simulink model "MSupGesamt"  (R2018b)
settings: Solver=FixedStepDiscrete  StartTime=0.0  StopTime=10.0  RelTol=1e-3  EnableMultiTasking=on
libraries: commutil2 x12, c280xlib x10, c2833xlib x9, c2000lib x1
(part 1 of 2)
settings Model: ExtModeTrigDuration=8  Creator=User  LastModifiedBy=ulvqy
settings SolverCC: AutoInsertRateTranBlk=on
settings DataIOCC: LimitDataPoints=on  SaveFormat=Array  SaveOutput=off  SaveTime=off
settings OptimizationCC: DefaultUnderspecifiedDataType=single  ExpressionDepthLimit=2147483647  LifeSpan=1  MaxStackSize=512
settings DebuggingCC: UnderspecifiedInitializationDetection=Classic  MergeDetectMultiDrivingBlocksExec=none  SolverPrmCheckMsg=warning  StateNameClashWarn=warning  SFUnexpectedBacktrackingDiag=warning  SFNoUnconditionalDefaultTransitionDiag=warning  SFExecutionAtInitializationDiag=none
settings HardwareCC: ProdBitPerChar=16  ProdBitPerInt=16  ProdBitPerPointer=32  ProdBitPerSizeT=32  ProdBitPerPtrDiffT=32  ProdLargestAtomicInteger=Integer  ProdLargestAtomicFloat=None  ProdWordSize=16  ProdLongLongMode=on  ProdHWDeviceType=Texas Instruments->C2000  TargetBitPerChar=16  TargetBitPerInt=16  TargetLargestAtomicInteger=Integer  TargetIntDivRoundTo=Zero  TargetEndianess=LittleEndian  TargetWordSize=16  TargetHWDeviceType=Texas Instruments->C2000  ProdEqTarget=off
settings ModelReferenceCC: PropagateSignalLabelsOutOfModel=off
settings SFSimCC: SimCustomSourceCode="#include \"i2c_reset.c\""  SimCustomHeaderCode="#include \"i2c_reset.h\""  SimUseLocalCustomCode=off  MATLABDynamicMemAlloc=off
settings RTWCC: SystemTargetFile=ert.tlc  HardwareBoard=TI Delfino F2833x  TemplateMakefile=ert_default_tmf  RTWUseLocalCustomCode=off  RTWUseSimCustomCode=on  CustomSourceCode="#include \"i2c_reset.c\""  CustomHeaderCode="#include \"i2c_reset.h\""  Toolchain=Texas Instruments Code Composer Studio (C2000)
settings CodeAppCC: IgnoreCustomStorageClasses=off  CustomSymbolStrType=$N$R$M  StateflowObjectComments=on  InternalIdentifier=Classic
settings ERTTargetCC: CodeReplacementLibrary=TI C28x  MultiwordLength=2048  ParMdlRefBuildCompliant=off  CPPClassGenCompliant=off  ConvertIfToSwitch=off  SuppressUnreachableDefaultCases=off
settings ConfigComp: CovMetricSettings=dw  CovHtmlReporting=on  CovSaveCumulativeToWorkspaceVar=on  CovSaveSingleToWorkspaceVar=on  CovExternalEMLEnable=off

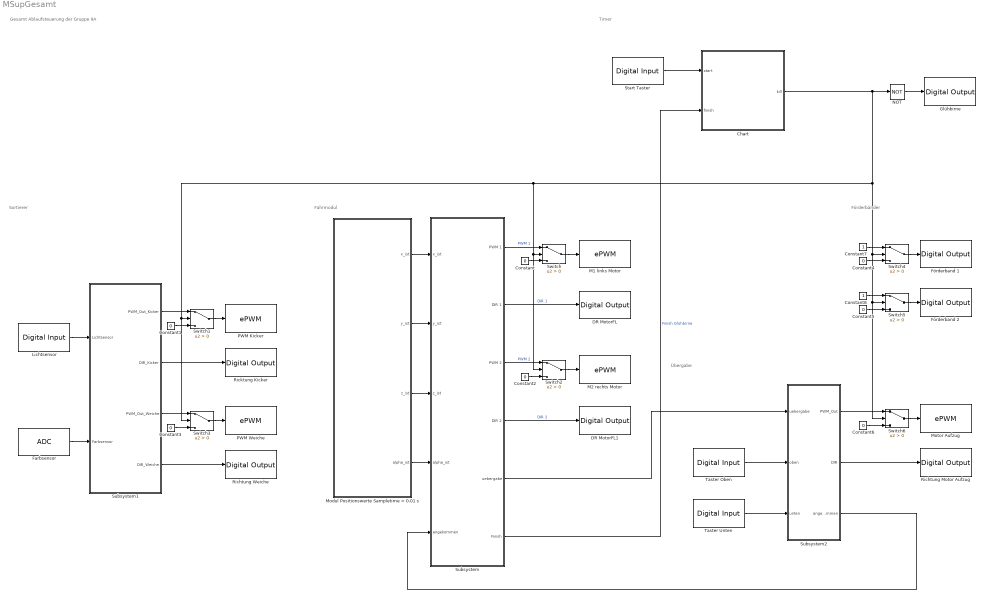
== system MSupGesamt ==
  note: Gesamt Ablaufsteuerung der Gruppe 9A
  note: Übergabe
  note: Timer
  note: Förderbänder
  note: Fahrmodul
  note: Sortierer
  Chart : Stateflow chart  TreatAsAtomicUnit=on
  Constant{,1..6} (7 alike) : Constant  Value=0
  Constant7 : Constant
  Constant8 : Constant
  DR MotorFL : c2833xlib/Digital Output  GPIO_Number=GPIO16~GPIO23  GPIO_Bit0=off  GPIO_BIT0_Toggle=off  GPIO_Bit1=off  GPIO_BIT1_Toggle=off  GPIO_Bit2=off  GPIO_BIT2_Toggle=off  GPIO_Bit3=off  GPIO_BIT3_Toggle=off  GPIO_Bit4=off  GPIO_BIT4_Toggle=off  GPIO_Bit5=on  GPIO_BIT5_Toggle=off  GPIO_Bit6=off  GPIO_BIT6_Toggle=off  GPIO_Bit7=off  GPIO_BIT7_Toggle=off
      settings: SourceProductName=Embedded Coder Support Package for Texas Instruments C2000 Processors  SourceProductBaseCode=TIC2000
  DR MotorFL1 : c2833xlib/Digital Output  GPIO_Number=GPIO16~GPIO23  GPIO_Bit0=off  GPIO_BIT0_Toggle=off  GPIO_Bit1=off  GPIO_BIT1_Toggle=off  GPIO_Bit2=off  GPIO_BIT2_Toggle=off  GPIO_Bit3=off  GPIO_BIT3_Toggle=off  GPIO_Bit4=on  GPIO_BIT4_Toggle=off  GPIO_Bit5=off  GPIO_BIT5_Toggle=off  GPIO_Bit6=off  GPIO_BIT6_Toggle=off  GPIO_Bit7=off  GPIO_BIT7_Toggle=off
      settings: SourceProductName=Embedded Coder Support Package for Texas Instruments C2000 Processors  SourceProductBaseCode=TIC2000
  Farbsensor : c280xlib/ADC  useModule=A  useMode=Sequential  sourceSOC=Software  sourceSOC1=Software  sourceSOC2=ePWMxB  xint2_ADCSOC=31  Ts=0.00002  dType=double  postInterrupt=off  numConversionsSingle=1  numConversionsDouble=1  conv0=ADCINA0  conv1=ADCINA1  conv2=ADCINA2  conv3=ADCINA3  conv4=ADCINA4  conv5=ADCINA5  conv6=ADCINA6  conv7=ADCINA7  conv8=ADCINB0  conv9=ADCINB1  conv10=ADCINB2  conv11=ADCINB3  conv12=ADCINB4  conv13=ADCINB5  conv14=ADCINB6  conv15=ADCINB7  convAB0=ADCINA0 and ADCINB0  convAB1=ADCINA1 and ADCINB1  convAB2=ADCINA2 and ADCINB2  convAB3=ADCINA3 and ADCINB3  convAB4=ADCINA4 and ADCINB4  convAB5=ADCINA5 and ADCINB5  convAB6=ADCINA6 and ADCINB6  convAB7=ADCINA7 and ADCINB7  convA0=ADCINA2  convA1=ADCINA1  convA2=ADCINA2  convA3=ADCINA3  convA4=ADCINA5  convA5=ADCINA5  convA6=ADCINA6  convA7=ADCINA7  convB0=ADCINB0  convB1=ADCINB1  convB2=ADCINB2  convB3=ADCINB3  convB4=ADCINB4  convB5=ADCINB5  convB6=ADCINB6  convB7=ADCINB7  c28xmultiPort=off  endma=off  chdma=1
      settings: SourceProductName=Embedded Coder Support Package for Texas Instruments C2000 Processors  SourceProductBaseCode=TIC2000
  Förderband 1 : c2833xlib/Digital Output  GPIO_Number=GPIO56~GPIO63  GPIO_Bit0=off  GPIO_BIT0_Toggle=off  GPIO_Bit1=off  GPIO_BIT1_Toggle=off  GPIO_Bit2=on  GPIO_BIT2_Toggle=off  GPIO_Bit3=off  GPIO_BIT3_Toggle=off  GPIO_Bit4=off  GPIO_BIT4_Toggle=off  GPIO_Bit5=off  GPIO_BIT5_Toggle=off  GPIO_Bit6=off  GPIO_BIT6_Toggle=off  GPIO_Bit7=off  GPIO_BIT7_Toggle=off
      settings: SourceProductName=Embedded Coder Support Package for Texas Instruments C2000 Processors  SourceProductBaseCode=TIC2000
  Förderband 2 : c2833xlib/Digital Output  GPIO_Number=GPIO56~GPIO63  GPIO_Bit0=off  GPIO_BIT0_Toggle=off  GPIO_Bit1=off  GPIO_BIT1_Toggle=off  GPIO_Bit2=off  GPIO_BIT2_Toggle=off  GPIO_Bit3=off  GPIO_BIT3_Toggle=off  GPIO_Bit4=off  GPIO_BIT4_Toggle=off  GPIO_Bit5=on  GPIO_BIT5_Toggle=off  GPIO_Bit6=off  GPIO_BIT6_Toggle=off  GPIO_Bit7=off  GPIO_BIT7_Toggle=off
      settings: SourceProductName=Embedded Coder Support Package for Texas Instruments C2000 Processors  SourceProductBaseCode=TIC2000
  Glühbirne : c2833xlib/Digital Output  GPIO_Number=GPIO56~GPIO63  GPIO_Bit0=off  GPIO_BIT0_Toggle=off  GPIO_Bit1=off  GPIO_BIT1_Toggle=off  GPIO_Bit2=off  GPIO_BIT2_Toggle=off  GPIO_Bit3=off  GPIO_BIT3_Toggle=off  GPIO_Bit4=on  GPIO_BIT4_Toggle=off  GPIO_Bit5=off  GPIO_BIT5_Toggle=off  GPIO_Bit6=off  GPIO_BIT6_Toggle=off  GPIO_Bit7=off  GPIO_BIT7_Toggle=off
      settings: SourceProductName=Embedded Coder Support Package for Texas Instruments C2000 Processors  SourceProductBaseCode=TIC2000
  Lichtsensor : c280xlib/Digital Input  GPIO_Number=GPIO24~GPIO31  GPIO_Bit0=off  GPIO_Bit1=on  GPIO_Bit2=off  GPIO_Bit3=off  GPIO_Bit4=off  GPIO_Bit5=off  GPIO_Bit6=off  GPIO_Bit7=off  sampleTime=0.1  dataType=auto  GPIO_Bit0_Qualification=Sync to SYSCLKOUT  GPIO_Bit1_Qualification=Sync to SYSCLKOUT  GPIO_Bit2_Qualification=Sync to SYSCLKOUT  GPIO_Bit3_Qualification=Sync to SYSCLKOUT  GPIO_Bit4_Qualification=Sync to SYSCLKOUT  GPIO_Bit5_Qualification=Sync to SYSCLKOUT  GPIO_Bit6_Qualification=Sync to SYSCLKOUT  GPIO_Bit7_Qualification=Sync to SYSCLKOUT  Qualification_Period=-1
      settings: SourceProductName=Embedded Coder Support Package for Texas Instruments C2000 Processors  SourceProductBaseCode=TIC2000
  M1 links Motor : c280xlib/ePWM  checkMode=off  useModule=ePWM2  periodUnits=Clock cycles  timerSource=Specify via dialog  timerPeriod_clk=64000  timerPeriod_sec=0.0001  tbshadow=Counter equals to zero  countingMode=Up  phaseActiveEnable=Disable  phaseDirection=Count down after sync  phaseActive=0  synchronizationEnable=off  synchronizationOption=Disable  clockPrescale=1  HSclockPrescale=1  ePWMxAStatus=on  CMPAUnits=Clock cycles  CMPASource=Specify via dialog  CMPAValue_per=50  CMPAValue_clk=32000  enCMPAshadow=Counter equals to zero  ePWMxAactionLogic1=Set  ePWMxAactionLogic2=Clear  ePWMxAactionLogic3=Clear  ePWMxAactionLogic4=Set  ePWMxAactionLogic5=Do nothing  ePWMxAactionLogic6=Do nothing  ePWMxALoadMode=Load on counter equals to zero (CTR=Zero)  ePWMxACSFenable=off  ePWMxACSFvalue=Forcing disable  ePWMxASFreload=Zero  enHRPWM=off  HRPWM_LoadMode=Counter equals to zero (CTR=ZERO)  HRPWM_CTLMode=Phase control mode  HRPWM_EDGMode=Both edge  enSFO=on  ePWMxBStatus=on  CMPBUnits=Percentages  CMPBSource=Input port  CMPBValue_per=0  CMPBValue_clk=32000  enCMPBshadow=Counter equals to zero  ePWMxBactionLogic1=Do nothing  ePWMxBactionLogic2=Set  ePWMxBactionLogic3=Do nothing  ePWMxBactionLogic4=Do nothing  ePWMxBactionLogic5=Clear  ePWMxBactionLogic6=Do nothing  ePWMxBLoadMode=Load on counter equals to zero (CTR=Zero)  ePWMxBCSFenable=off  ePWMxBCSFvalue=Forcing disable  ePWMxBSFreload=Zero  enableDBePWMxA=off  enableDBePWMxB=off  DBpolarity=Active high (AH)  DBedgeDelay=Positive  DBSource_ePWMxA=ePWMxA  DBSource_ePWMxB=ePWMxA  DBperiodSource=Specify via dialog  REDperiod=0  FEDperiod=0  adcstartModuleA=off  adcrequestEventA=First event  adcstartEventA=Counter equals to zero (CTR=Zero)  adcstartModuleB=off  adcrequestEventB=First event  adcstartEventB=Counter equals to zero (CTR=Zero)  intEn=off  intPrd=First event  intSel=Counter equals to zero (CTR=Zero)  chopperEnable=off  chopperFrequency=1  chopperFirstwidth=1  chopperDuty=12.5%  tripZonesource=Specify via dialog  tzselOSHT1=off  tzselOSHT2=off  tzselOSHT3=off  tzselOSHT4=off  tzselOSHT5=off  tzselOSHT6=off  tzselCBC1=off  tzselCBC2=off  tzselCBC3=off  tzselCBC4=off  tzselCBC5=off  tzselCBC6=off  enTzOstIntr=off  enTzCbcIntr=off  ePWMxAforced=No action  ePWMxBforced=No action  timerPeriod=-1  ePWMxAValue=0  ePWMxBValue=0  tripZoneoption=One-shot trip (OSHT)
      settings: SourceProductName=Embedded Coder Support Package for Texas Instruments C2000 Processors  SourceProductBaseCode=TIC2000
  M2 rechts Motor : c280xlib/ePWM  checkMode=off  useModule=ePWM1  periodUnits=Clock cycles  timerSource=Specify via dialog  timerPeriod_clk=64000  timerPeriod_sec=0.0001  tbshadow=Counter equals to zero  countingMode=Up  phaseActiveEnable=Disable  phaseDirection=Count down after sync  phaseActive=0  synchronizationEnable=off  synchronizationOption=Disable  clockPrescale=1  HSclockPrescale=1  ePWMxAStatus=on  CMPAUnits=Clock cycles  CMPASource=Specify via dialog  CMPAValue_per=50  CMPAValue_clk=32000  enCMPAshadow=Counter equals to zero  ePWMxAactionLogic1=Set  ePWMxAactionLogic2=Clear  ePWMxAactionLogic3=Clear  ePWMxAactionLogic4=Set  ePWMxAactionLogic5=Do nothing  ePWMxAactionLogic6=Do nothing  ePWMxALoadMode=Load on counter equals to zero (CTR=Zero)  ePWMxACSFenable=off  ePWMxACSFvalue=Forcing disable  ePWMxASFreload=Zero  enHRPWM=off  HRPWM_LoadMode=Counter equals to zero (CTR=ZERO)  HRPWM_CTLMode=Phase control mode  HRPWM_EDGMode=Both edge  enSFO=on  ePWMxBStatus=on  CMPBUnits=Percentages  CMPBSource=Input port  CMPBValue_per=0  CMPBValue_clk=32000  enCMPBshadow=Counter equals to zero  ePWMxBactionLogic1=Do nothing  ePWMxBactionLogic2=Set  ePWMxBactionLogic3=Do nothing  ePWMxBactionLogic4=Do nothing  ePWMxBactionLogic5=Clear  ePWMxBactionLogic6=Do nothing  ePWMxBLoadMode=Load on counter equals to zero (CTR=Zero)  ePWMxBCSFenable=off  ePWMxBCSFvalue=Forcing disable  ePWMxBSFreload=Zero  enableDBePWMxA=off  enableDBePWMxB=off  DBpolarity=Active high (AH)  DBedgeDelay=Positive  DBSource_ePWMxA=ePWMxA  DBSource_ePWMxB=ePWMxA  DBperiodSource=Specify via dialog  REDperiod=0  FEDperiod=0  adcstartModuleA=off  adcrequestEventA=First event  adcstartEventA=Counter equals to zero (CTR=Zero)  adcstartModuleB=off  adcrequestEventB=First event  adcstartEventB=Counter equals to zero (CTR=Zero)  intEn=off  intPrd=First event  intSel=Counter equals to zero (CTR=Zero)  chopperEnable=off  chopperFrequency=1  chopperFirstwidth=1  chopperDuty=12.5%  tripZonesource=Specify via dialog  tzselOSHT1=off  tzselOSHT2=off  tzselOSHT3=off  tzselOSHT4=off  tzselOSHT5=off  tzselOSHT6=off  tzselCBC1=off  tzselCBC2=off  tzselCBC3=off  tzselCBC4=off  tzselCBC5=off  tzselCBC6=off  enTzOstIntr=off  enTzCbcIntr=off  ePWMxAforced=No action  ePWMxBforced=No action  timerPeriod=-1  ePWMxAValue=0  ePWMxBValue=0  tripZoneoption=One-shot trip (OSHT)
      settings: SourceProductName=Embedded Coder Support Package for Texas Instruments C2000 Processors  SourceProductBaseCode=TIC2000
  Modul Positionswerte Sampletime = 0.01 s : Subsystem
  Motor Aufzug : c280xlib/ePWM  checkMode=off  useModule=ePWM3  periodUnits=Clock cycles  timerSource=Specify via dialog  timerPeriod_clk=64000  timerPeriod_sec=0.0001  tbshadow=Counter equals to zero  countingMode=Up  phaseActiveEnable=Disable  phaseDirection=Count down after sync  phaseActive=0  synchronizationEnable=off  synchronizationOption=Disable  clockPrescale=1  HSclockPrescale=1  ePWMxAStatus=on  CMPAUnits=Clock cycles  CMPASource=Specify via dialog  CMPAValue_per=50  CMPAValue_clk=32000  enCMPAshadow=Counter equals to zero  ePWMxAactionLogic1=Set  ePWMxAactionLogic2=Clear  ePWMxAactionLogic3=Clear  ePWMxAactionLogic4=Set  ePWMxAactionLogic5=Do nothing  ePWMxAactionLogic6=Do nothing  ePWMxALoadMode=Load on counter equals to zero (CTR=Zero)  ePWMxACSFenable=off  ePWMxACSFvalue=Forcing disable  ePWMxASFreload=Zero  enHRPWM=off  HRPWM_LoadMode=Counter equals to zero (CTR=ZERO)  HRPWM_CTLMode=Phase control mode  HRPWM_EDGMode=Both edge  enSFO=on  ePWMxBStatus=on  CMPBUnits=Percentages  CMPBSource=Input port  CMPBValue_per=0  CMPBValue_clk=32000  enCMPBshadow=Counter equals to zero  ePWMxBactionLogic1=Do nothing  ePWMxBactionLogic2=Set  ePWMxBactionLogic3=Do nothing  ePWMxBactionLogic4=Do nothing  ePWMxBactionLogic5=Clear  ePWMxBactionLogic6=Do nothing  ePWMxBLoadMode=Load on counter equals to zero (CTR=Zero)  ePWMxBCSFenable=off  ePWMxBCSFvalue=Forcing disable  ePWMxBSFreload=Zero  enableDBePWMxA=off  enableDBePWMxB=off  DBpolarity=Active high (AH)  DBedgeDelay=Positive  DBSource_ePWMxA=ePWMxA  DBSource_ePWMxB=ePWMxA  DBperiodSource=Specify via dialog  REDperiod=0  FEDperiod=0  adcstartModuleA=off  adcrequestEventA=First event  adcstartEventA=Counter equals to zero (CTR=Zero)  adcstartModuleB=off  adcrequestEventB=First event  adcstartEventB=Counter equals to zero (CTR=Zero)  intEn=off  intPrd=First event  intSel=Counter equals to zero (CTR=Zero)  chopperEnable=off  chopperFrequency=1  chopperFirstwidth=1  chopperDuty=12.5%  tripZonesource=Specify via dialog  tzselOSHT1=off  tzselOSHT2=off  tzselOSHT3=off  tzselOSHT4=off  tzselOSHT5=off  tzselOSHT6=off  tzselCBC1=off  tzselCBC2=off  tzselCBC3=off  tzselCBC4=off  tzselCBC5=off  tzselCBC6=off  enTzOstIntr=off  enTzCbcIntr=off  ePWMxAforced=No action  ePWMxBforced=No action  timerPeriod=-1  ePWMxAValue=0  ePWMxBValue=0  tripZoneoption=One-shot trip (OSHT)
      settings: SourceProductName=Embedded Coder Support Package for Texas Instruments C2000 Processors  SourceProductBaseCode=TIC2000
  NOT : Logic  Operator=NOT  IconShape=distinctive  AllPortsSameDT=off  OutDataTypeStr=boolean
  PWM Kicker : c280xlib/ePWM  checkMode=off  useModule=ePWM5  periodUnits=Clock cycles  timerSource=Specify via dialog  timerPeriod_clk=64000  timerPeriod_sec=0.0001  tbshadow=Counter equals to zero  countingMode=Up  phaseActiveEnable=Disable  phaseDirection=Count down after sync  phaseActive=0  synchronizationEnable=off  synchronizationOption=Disable  clockPrescale=1  HSclockPrescale=1  ePWMxAStatus=off  CMPAUnits=Clock cycles  CMPASource=Specify via dialog  CMPAValue_per=50  CMPAValue_clk=32000  enCMPAshadow=Counter equals to zero  ePWMxAactionLogic1=Do nothing  ePWMxAactionLogic2=Clear  ePWMxAactionLogic3=Set  ePWMxAactionLogic4=Do nothing  ePWMxAactionLogic5=Do nothing  ePWMxAactionLogic6=Do nothing  ePWMxALoadMode=Load on counter equals to zero (CTR=Zero)  ePWMxACSFenable=off  ePWMxACSFvalue=Forcing disable  ePWMxASFreload=Zero  enHRPWM=off  HRPWM_LoadMode=Counter equals to zero (CTR=ZERO)  HRPWM_CTLMode=Phase control mode  HRPWM_EDGMode=Both edge  enSFO=on  ePWMxBStatus=on  CMPBUnits=Percentages  CMPBSource=Input port  CMPBValue_per=0  CMPBValue_clk=32000  enCMPBshadow=Counter equals to zero  ePWMxBactionLogic1=Do nothing  ePWMxBactionLogic2=Set  ePWMxBactionLogic3=Do nothing  ePWMxBactionLogic4=Do nothing  ePWMxBactionLogic5=Clear  ePWMxBactionLogic6=Do nothing  ePWMxBLoadMode=Load on counter equals to zero (CTR=Zero)  ePWMxBCSFenable=off  ePWMxBCSFvalue=Forcing disable  ePWMxBSFreload=Zero  enableDBePWMxA=off  enableDBePWMxB=off  DBpolarity=Active high (AH)  DBedgeDelay=Positive  DBSource_ePWMxA=ePWMxA  DBSource_ePWMxB=ePWMxA  DBperiodSource=Specify via dialog  REDperiod=0  FEDperiod=0  adcstartModuleA=off  adcrequestEventA=First event  adcstartEventA=Counter equals to zero (CTR=Zero)  adcstartModuleB=off  adcrequestEventB=First event  adcstartEventB=Counter equals to zero (CTR=Zero)  intEn=off  intPrd=First event  intSel=Counter equals to zero (CTR=Zero)  chopperEnable=off  chopperFrequency=1  chopperFirstwidth=1  chopperDuty=12.5%  tripZonesource=Specify via dialog  tzselOSHT1=off  tzselOSHT2=off  tzselOSHT3=off  tzselOSHT4=off  tzselOSHT5=off  tzselOSHT6=off  tzselCBC1=off  tzselCBC2=off  tzselCBC3=off  tzselCBC4=off  tzselCBC5=off  tzselCBC6=off  enTzOstIntr=off  enTzCbcIntr=off  ePWMxAforced=No action  ePWMxBforced=No action  timerPeriod=-1  ePWMxAValue=0  ePWMxBValue=0  tripZoneoption=One-shot trip (OSHT)
      settings: SourceProductName=Embedded Coder Support Package for Texas Instruments C2000 Processors  SourceProductBaseCode=TIC2000
  PWM Weiche : c280xlib/ePWM  checkMode=off  useModule=ePWM6  periodUnits=Clock cycles  timerSource=Specify via dialog  timerPeriod_clk=64000  timerPeriod_sec=0.0001  tbshadow=Counter equals to zero  countingMode=Up  phaseActiveEnable=Disable  phaseDirection=Count down after sync  phaseActive=0  synchronizationEnable=off  synchronizationOption=Disable  clockPrescale=1  HSclockPrescale=1  ePWMxAStatus=off  CMPAUnits=Clock cycles  CMPASource=Specify via dialog  CMPAValue_per=50  CMPAValue_clk=32000  enCMPAshadow=Counter equals to zero  ePWMxAactionLogic1=Do nothing  ePWMxAactionLogic2=Clear  ePWMxAactionLogic3=Set  ePWMxAactionLogic4=Do nothing  ePWMxAactionLogic5=Do nothing  ePWMxAactionLogic6=Do nothing  ePWMxALoadMode=Load on counter equals to zero (CTR=Zero)  ePWMxACSFenable=off  ePWMxACSFvalue=Forcing disable  ePWMxASFreload=Zero  enHRPWM=off  HRPWM_LoadMode=Counter equals to zero (CTR=ZERO)  HRPWM_CTLMode=Phase control mode  HRPWM_EDGMode=Both edge  enSFO=on  ePWMxBStatus=on  CMPBUnits=Percentages  CMPBSource=Input port  CMPBValue_per=0  CMPBValue_clk=32000  enCMPBshadow=Counter equals to zero  ePWMxBactionLogic1=Do nothing  ePWMxBactionLogic2=Set  ePWMxBactionLogic3=Do nothing  ePWMxBactionLogic4=Do nothing  ePWMxBactionLogic5=Clear  ePWMxBactionLogic6=Do nothing  ePWMxBLoadMode=Load on counter equals to zero (CTR=Zero)  ePWMxBCSFenable=off  ePWMxBCSFvalue=Forcing disable  ePWMxBSFreload=Zero  enableDBePWMxA=off  enableDBePWMxB=off  DBpolarity=Active high (AH)  DBedgeDelay=Positive  DBSource_ePWMxA=ePWMxA  DBSource_ePWMxB=ePWMxA  DBperiodSource=Specify via dialog  REDperiod=0  FEDperiod=0  adcstartModuleA=off  adcrequestEventA=First event  adcstartEventA=Counter equals to zero (CTR=Zero)  adcstartModuleB=off  adcrequestEventB=First event  adcstartEventB=Counter equals to zero (CTR=Zero)  intEn=off  intPrd=First event  intSel=Counter equals to zero (CTR=Zero)  chopperEnable=off  chopperFrequency=1  chopperFirstwidth=1  chopperDuty=12.5%  tripZonesource=Specify via dialog  tzselOSHT1=off  tzselOSHT2=off  tzselOSHT3=off  tzselOSHT4=off  tzselOSHT5=off  tzselOSHT6=off  tzselCBC1=off  tzselCBC2=off  tzselCBC3=off  tzselCBC4=off  tzselCBC5=off  tzselCBC6=off  enTzOstIntr=off  enTzCbcIntr=off  ePWMxAforced=No action  ePWMxBforced=No action  timerPeriod=-1  ePWMxAValue=0  ePWMxBValue=0  tripZoneoption=One-shot trip (OSHT)
      settings: SourceProductName=Embedded Coder Support Package for Texas Instruments C2000 Processors  SourceProductBaseCode=TIC2000
  Richtung Motor Aufzug : c2833xlib/Digital Output  GPIO_Number=GPIO16~GPIO23  GPIO_Bit0=off  GPIO_BIT0_Toggle=off  GPIO_Bit1=on  GPIO_BIT1_Toggle=off  GPIO_Bit2=off  GPIO_BIT2_Toggle=off  GPIO_Bit3=off  GPIO_BIT3_Toggle=off  GPIO_Bit4=off  GPIO_BIT4_Toggle=off  GPIO_Bit5=off  GPIO_BIT5_Toggle=off  GPIO_Bit6=off  GPIO_BIT6_Toggle=off  GPIO_Bit7=off  GPIO_BIT7_Toggle=off
      settings: SourceProductName=Embedded Coder Support Package for Texas Instruments C2000 Processors  SourceProductBaseCode=TIC2000
  Richtung Weiche : c2833xlib/Digital Output  GPIO_Number=GPIO16~GPIO23  GPIO_Bit0=on  GPIO_BIT0_Toggle=off  GPIO_Bit1=off  GPIO_BIT1_Toggle=off  GPIO_Bit2=off  GPIO_BIT2_Toggle=off  GPIO_Bit3=off  GPIO_BIT3_Toggle=off  GPIO_Bit4=off  GPIO_BIT4_Toggle=off  GPIO_Bit5=off  GPIO_BIT5_Toggle=off  GPIO_Bit6=off  GPIO_BIT6_Toggle=off  GPIO_Bit7=off  GPIO_BIT7_Toggle=off
      settings: SourceProductName=Embedded Coder Support Package for Texas Instruments C2000 Processors  SourceProductBaseCode=TIC2000
  Ricktung Kicker : c2833xlib/Digital Output  GPIO_Number=GPIO8~GPIO15  GPIO_Bit0=off  GPIO_BIT0_Toggle=off  GPIO_Bit1=off  GPIO_BIT1_Toggle=off  GPIO_Bit2=off  GPIO_BIT2_Toggle=off  GPIO_Bit3=off  GPIO_BIT3_Toggle=off  GPIO_Bit4=off  GPIO_BIT4_Toggle=off  GPIO_Bit5=off  GPIO_BIT5_Toggle=off  GPIO_Bit6=off  GPIO_BIT6_Toggle=off  GPIO_Bit7=on  GPIO_BIT7_Toggle=off
      settings: SourceProductName=Embedded Coder Support Package for Texas Instruments C2000 Processors  SourceProductBaseCode=TIC2000
  Start Taster : c2833xlib/Digital Input  GPIO_Number=GPIO24~GPIO31  GPIO_Bit0=off  GPIO_Bit1=off  GPIO_Bit2=off  GPIO_Bit3=off  GPIO_Bit4=off  GPIO_Bit5=off  GPIO_Bit6=off  GPIO_Bit7=on  sampleTime=0.1  dataType=auto  GPIO_Bit0_Qualification=Sync to SYSCLKOUT  GPIO_Bit1_Qualification=Sync to SYSCLKOUT  GPIO_Bit2_Qualification=Sync to SYSCLKOUT  GPIO_Bit3_Qualification=Sync to SYSCLKOUT  GPIO_Bit4_Qualification=Sync to SYSCLKOUT  GPIO_Bit5_Qualification=Sync to SYSCLKOUT  GPIO_Bit6_Qualification=Sync to SYSCLKOUT  GPIO_Bit7_Qualification=Sync to SYSCLKOUT  Qualification_Period=-1
      settings: SourceProductName=Embedded Coder Support Package for Texas Instruments C2000 Processors  SourceProductBaseCode=TIC2000
  Subsystem : Subsystem
  Subsystem1 : Subsystem
  Subsystem2 : Subsystem
  Switch{,1..6} (7 alike) : Switch  Criteria=u2 > Threshold
  Taster Oben : c280xlib/Digital Input  GPIO_Number=GPIO24~GPIO31  GPIO_Bit0=off  GPIO_Bit1=off  GPIO_Bit2=on  GPIO_Bit3=off  GPIO_Bit4=off  GPIO_Bit5=off  GPIO_Bit6=off  GPIO_Bit7=off  sampleTime=0.1  dataType=auto  GPIO_Bit0_Qualification=Sync to SYSCLKOUT  GPIO_Bit1_Qualification=Sync to SYSCLKOUT  GPIO_Bit2_Qualification=Sync to SYSCLKOUT  GPIO_Bit3_Qualification=Sync to SYSCLKOUT  GPIO_Bit4_Qualification=Sync to SYSCLKOUT  GPIO_Bit5_Qualification=Sync to SYSCLKOUT  GPIO_Bit6_Qualification=Sync to SYSCLKOUT  GPIO_Bit7_Qualification=Sync to SYSCLKOUT  Qualification_Period=-1
      settings: SourceProductName=Embedded Coder Support Package for Texas Instruments C2000 Processors  SourceProductBaseCode=TIC2000
  Taster Unten : c280xlib/Digital Input  GPIO_Number=GPIO24~GPIO31  GPIO_Bit0=off  GPIO_Bit1=off  GPIO_Bit2=off  GPIO_Bit3=on  GPIO_Bit4=off  GPIO_Bit5=off  GPIO_Bit6=off  GPIO_Bit7=off  sampleTime=0.1  dataType=auto  GPIO_Bit0_Qualification=Sync to SYSCLKOUT  GPIO_Bit1_Qualification=Sync to SYSCLKOUT  GPIO_Bit2_Qualification=Sync to SYSCLKOUT  GPIO_Bit3_Qualification=Sync to SYSCLKOUT  GPIO_Bit4_Qualification=Sync to SYSCLKOUT  GPIO_Bit5_Qualification=Sync to SYSCLKOUT  GPIO_Bit6_Qualification=Sync to SYSCLKOUT  GPIO_Bit7_Qualification=Sync to SYSCLKOUT  Qualification_Period=-1
      settings: SourceProductName=Embedded Coder Support Package for Texas Instruments C2000 Processors  SourceProductBaseCode=TIC2000
  wires:
  Subsystem1/2(DIR_Kicker) -> Ricktung Kicker/1
  Subsystem1/3(PWM_Out_Weiche) -> Switch3/1
  Lichtsensor/1 -> Subsystem1/1(Lichtsensor)
  Subsystem1/4(DIR_Weiche) -> Richtung Weiche/1
  Subsystem1/1(PWM_Out_Kicker) -> Switch1/1
  Modul Positionswerte Sampletime = 0.01 s/2(y_ist) -> Subsystem/2(y_ist)
  Subsystem/3(PWM 2) -> Switch2/1  "PWM 2"
  Subsystem/6(Finish) -> Chart/2(finish)  "Finish Glühbirne"
  Subsystem/4("DIR 2 ") -> DR MotorFL1/1  "DIR 2"
  Subsystem/1(PWM 1) -> Switch/1  "PWM 1"
  Modul Positionswerte Sampletime = 0.01 s/1(x_ist) -> Subsystem/1(x_ist)
  Modul Positionswerte Sampletime = 0.01 s/4(alpha_ist) -> Subsystem/4(alpha_ist)
  Subsystem/2("DIR 1 ") -> DR MotorFL/1  "DIR 1"
  Modul Positionswerte Sampletime = 0.01 s/3(z_ist) -> Subsystem/3(z_ist)
  Farbsensor/1 -> Subsystem1/2(Farbsensor)
  Switch/1 -> M1 links Motor/1
  Constant/1 -> Switch/3
  Constant2/1 -> Switch2/3
  Switch2/1 -> M2 rechts Motor/1
  Constant1/1 -> Switch1/3
  Constant3/1 -> Switch3/3
  Switch1/1 -> PWM Kicker/1
  Switch3/1 -> PWM Weiche/1
  Constant4/1 -> Switch4/3
  Switch4/1 -> Förderband 1/1
  Constant5/1 -> Switch5/3
  Switch5/1 -> Förderband 2/1
  Constant6/1 -> Switch6/3
  Switch6/1 -> Motor Aufzug/1
  Chart/1(kill) -> Switch1/2, Switch3/2, Switch2/2, Switch/2, Switch6/2, Switch5/2, Switch4/2, NOT/1
  Constant7/1 -> Switch4/1
  Constant8/1 -> Switch5/1
  Start Taster/1 -> Chart/1(start)
  Subsystem2/1(PWM_Out) -> Switch6/1
  Subsystem/5(uebergabe) -> Subsystem2/1(uebergabe)
  Subsystem2/2(DIR) -> Richtung Motor Aufzug/1
  Taster Oben/1 -> Subsystem2/2(oben)
  Taster Unten/1 -> Subsystem2/3(unten)
  Subsystem2/3(angekommen) -> Subsystem/5(angekommen)
  NOT/1 -> Glühbirne/1

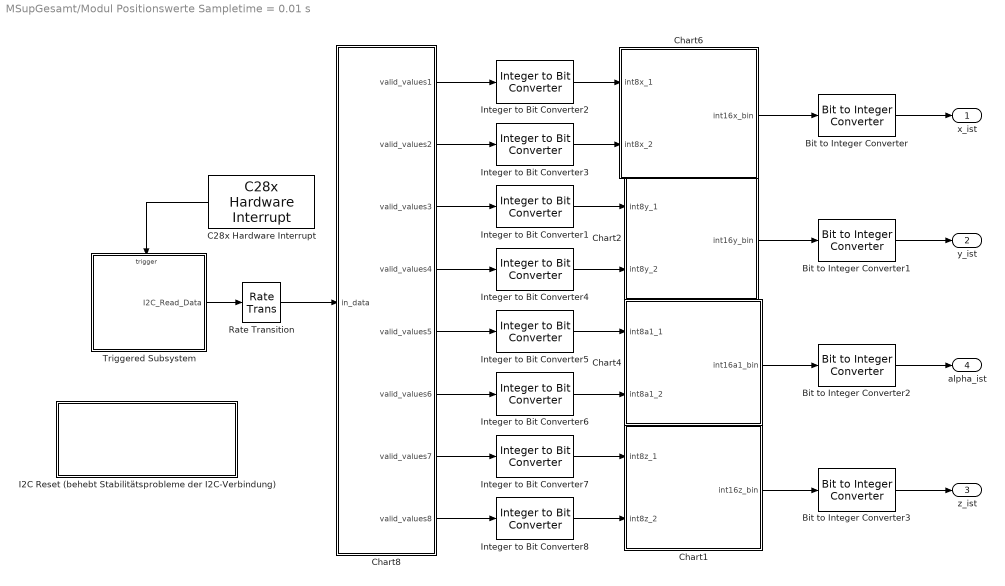
== system MSupGesamt/Modul Positionswerte Sampletime = 0.01 s ==
  Bit to Integer Converter{,1..3} (4 alike) : commutil2/Bit to Integer Converter  nbits=16  bitOrder=MSB first  signedOutputValues=Signed  outDtype=Inherit via internal rule  outDtypeSigned=Inherit via internal rule
      settings: SourceProductName=Communications Toolbox
  C28x Hardware Interrupt : c2000lib/Scheduling/C28x Hardware Interrupt  irqnumbers=8  pienumbers=2  irqpriorities=30  irqpreempts=0  showinput=off  dspchiptype=C280X
      settings: SourceProductName=Embedded Coder Support Package for Texas Instruments C2000 Processors  SourceProductBaseCode=TIC2000
  Chart1 : Stateflow chart  TreatAsAtomicUnit=on
  Chart2 : Stateflow chart  TreatAsAtomicUnit=on
  Chart4 : Stateflow chart  TreatAsAtomicUnit=on
  Chart6 : Stateflow chart  TreatAsAtomicUnit=on
  Chart8 : Stateflow chart  TreatAsAtomicUnit=on
  I2C Reset (behebt Stabilitätsprobleme der I2C-Verbindung) : Subsystem
  Integer to Bit Converter{1..8} (8 alike) : commutil2/Integer to Bit Converter  nbits=8  signedInputValues=Unsigned  bitOrder=MSB first  outDtype=uint8
      settings: SourceProductName=Communications Toolbox
  Rate Transition : RateTransition  Deterministic=off  OutPortSampleTime=0.01
  Triggered Subsystem : Subsystem  TreatAsAtomicUnit=on
  x_ist : Outport
  y_ist : Outport  Port=2
  z_ist : Outport  Port=3
  alpha_ist : Outport  Port=4
  wires:
  Integer to Bit Converter7/1 -> Chart1/1(int8z_1)
  Integer to Bit Converter8/1 -> Chart1/2(int8z_2)
  Chart8/7(valid_values7) -> Integer to Bit Converter7/1
  Chart8/8(valid_values8) -> Integer to Bit Converter8/1
  Bit to Integer Converter3/1 -> z_ist/1
  Triggered Subsystem/1(I2C_Read_Data) -> Rate Transition/1
  Chart1/1(int16z_bin) -> Bit to Integer Converter3/1
  Chart4/1(int16a1_bin) -> Bit to Integer Converter2/1
  Chart8/6(valid_values6) -> Integer to Bit Converter6/1
  Bit to Integer Converter2/1 -> alpha_ist/1
  Bit to Integer Converter/1 -> x_ist/1
  Integer to Bit Converter6/1 -> Chart4/2(int8a1_2)
  Integer to Bit Converter5/1 -> Chart4/1(int8a1_1)
  Bit to Integer Converter1/1 -> y_ist/1
  Integer to Bit Converter4/1 -> Chart2/2(int8y_2)
  Integer to Bit Converter2/1 -> Chart6/1(int8x_1)
  Integer to Bit Converter1/1 -> Chart2/1(int8y_1)
  Chart6/1(int16x_bin) -> Bit to Integer Converter/1
  Integer to Bit Converter3/1 -> Chart6/2(int8x_2)
  Chart8/3(valid_values3) -> Integer to Bit Converter1/1
  Chart8/1(valid_values1) -> Integer to Bit Converter2/1
  Chart2/1(int16y_bin) -> Bit to Integer Converter1/1
  Chart8/4(valid_values4) -> Integer to Bit Converter4/1
  Chart8/2(valid_values2) -> Integer to Bit Converter3/1
  Chart8/5(valid_values5) -> Integer to Bit Converter5/1
  C28x Hardware Interrupt/1 -> Triggered Subsystem/Trigger
  Rate Transition/1 -> Chart8/1(in_data)

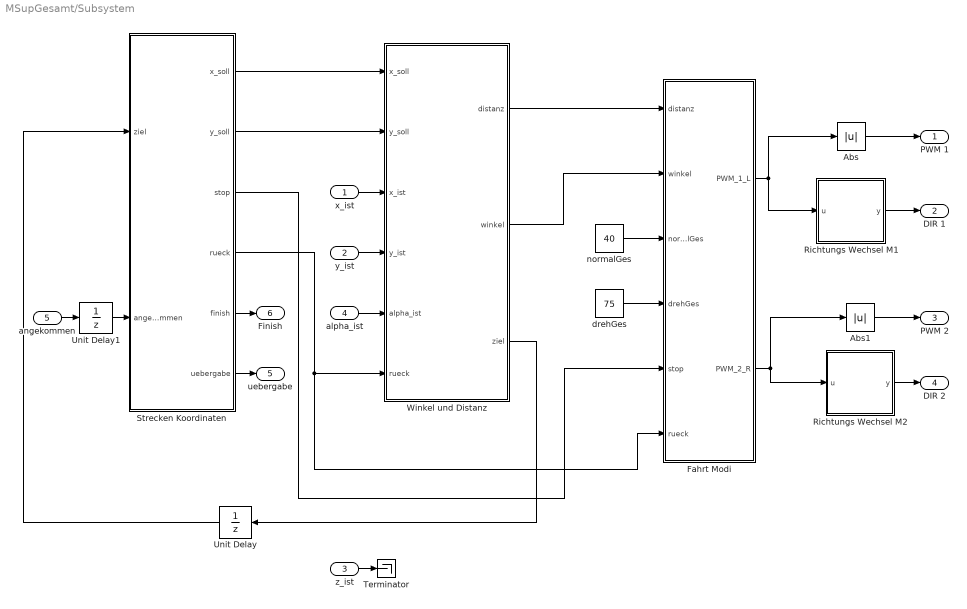
== system MSupGesamt/Subsystem ==
  x_ist : Inport
  y_ist : Inport  Port=2
  z_ist : Inport  Port=3
  alpha_ist : Inport  Port=4
  angekommen : Inport  Port=5
  Abs : Abs
  Abs1 : Abs
  Fahrt Modi : Stateflow chart  TreatAsAtomicUnit=on
  "Richtungs Wechsel M1 " : MATLAB Function  TreatAsAtomicUnit=on
  Richtungs Wechsel M2 : MATLAB Function  TreatAsAtomicUnit=on
  Strecken Koordinaten : Stateflow chart  TreatAsAtomicUnit=on
  Terminator : Terminator
  Unit Delay : UnitDelay  SampleTime=-1
  Unit Delay1 : UnitDelay  SampleTime=-1
  Winkel und Distanz : MATLAB Function  TreatAsAtomicUnit=on
  "drehGes " : Constant  Value=75
  "normalGes " : Constant  Value=40
  PWM 1 : Outport
  "DIR 1 " : Outport  Port=2
  PWM 2 : Outport  Port=3
  "DIR 2 " : Outport  Port=4
  uebergabe : Outport  Port=5
  Finish : Outport  Port=6
  wires:
  z_ist/1 -> Terminator/1
  Abs/1 -> PWM 1/1
  Abs1/1 -> PWM 2/1
  "Richtungs Wechsel M1 "/1(y) -> "DIR 1 "/1
  Fahrt Modi/1(PWM_1_L) -> Abs/1, "Richtungs Wechsel M1 "/1(u)
  Richtungs Wechsel M2/1(y) -> "DIR 2 "/1
  Fahrt Modi/2(PWM_2_R) -> Abs1/1, Richtungs Wechsel M2/1(u)
  y_ist/1 -> Winkel und Distanz/4(y_ist)
  x_ist/1 -> Winkel und Distanz/3(x_ist)
  "normalGes "/1 -> Fahrt Modi/3(normalGes)
  "drehGes "/1 -> Fahrt Modi/4(drehGes)
  Winkel und Distanz/1(distanz) -> Fahrt Modi/1(distanz)
  Winkel und Distanz/2(winkel) -> Fahrt Modi/2(winkel)
  alpha_ist/1 -> Winkel und Distanz/5(alpha_ist)
  Strecken Koordinaten/1(x_soll) -> Winkel und Distanz/1(x_soll)
  Strecken Koordinaten/2(y_soll) -> Winkel und Distanz/2(y_soll)
  Winkel und Distanz/3(ziel) -> Unit Delay/1
  Unit Delay/1 -> Strecken Koordinaten/1(ziel)
  Strecken Koordinaten/3(stop) -> Fahrt Modi/5(stop)
  Strecken Koordinaten/4(rueck) -> Winkel und Distanz/6(rueck), Fahrt Modi/6(rueck)
  Strecken Koordinaten/5(finish) -> Finish/1
  Strecken Koordinaten/6(uebergabe) -> uebergabe/1
  angekommen/1 -> Unit Delay1/1
  Unit Delay1/1 -> Strecken Koordinaten/2(angekommen)

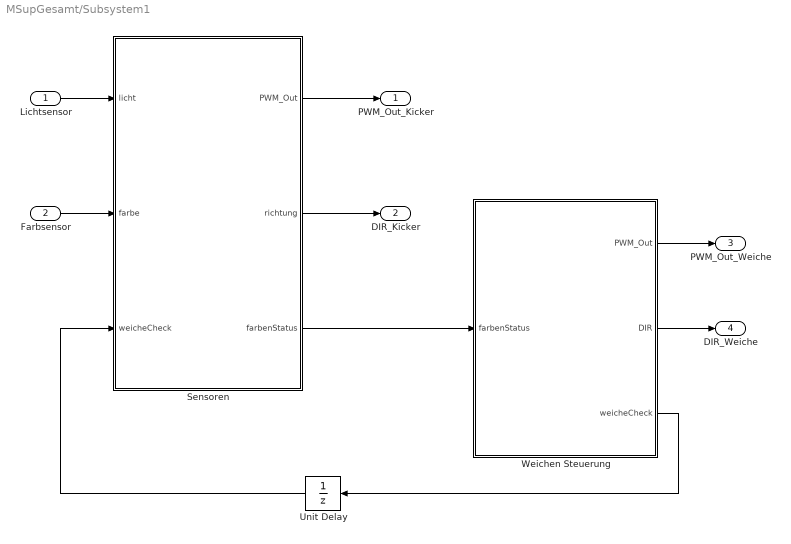
== system MSupGesamt/Subsystem1 ==
  Lichtsensor : Inport
  Farbsensor : Inport  Port=2
  Sensoren : Stateflow chart  TreatAsAtomicUnit=on
  Unit Delay : UnitDelay  SampleTime=-1
  Weichen Steuerung : Stateflow chart  TreatAsAtomicUnit=on
  PWM_Out_Kicker : Outport
  DIR_Kicker : Outport  Port=2
  PWM_Out_Weiche : Outport  Port=3
  DIR_Weiche : Outport  Port=4
  wires:
  Lichtsensor/1 -> Sensoren/1(licht)
  Farbsensor/1 -> Sensoren/2(farbe)
  Sensoren/1(PWM_Out) -> PWM_Out_Kicker/1
  Sensoren/2(richtung) -> DIR_Kicker/1
  Weichen Steuerung/1(PWM_Out) -> PWM_Out_Weiche/1
  Weichen Steuerung/2(DIR) -> DIR_Weiche/1
  Sensoren/3(farbenStatus) -> Weichen Steuerung/1(farbenStatus)
  Unit Delay/1 -> Sensoren/3(weicheCheck)
  Weichen Steuerung/3(weicheCheck) -> Unit Delay/1

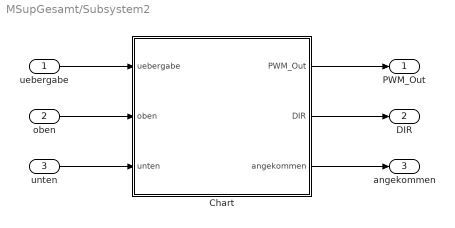
== system MSupGesamt/Subsystem2 ==
  uebergabe : Inport
  oben : Inport  Port=2
  unten : Inport  Port=3
  Chart : Stateflow chart  TreatAsAtomicUnit=on
  PWM_Out : Outport
  DIR : Outport  Port=2
  angekommen : Outport  Port=3
  wires:
  Chart/1(PWM_Out) -> PWM_Out/1
  Chart/2(DIR) -> DIR/1
  uebergabe/1 -> Chart/1(uebergabe)
  oben/1 -> Chart/2(oben)
  unten/1 -> Chart/3(unten)
  Chart/3(angekommen) -> angekommen/1

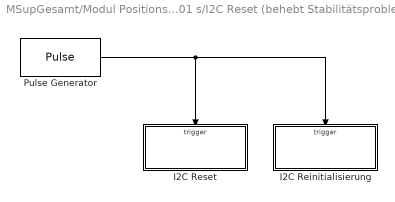
== system MSupGesamt/Modul Positionswerte Sampletime = 0.01 s/I2C Reset (behebt Stabilitätsprobleme der I2C-Verbindung) ==
  I2C Reinitialisierung : Subsystem  TreatAsAtomicUnit=on
  I2C Reset : Subsystem  TreatAsAtomicUnit=on
  Pulse Generator : DiscretePulseGenerator  Period=250  SampleTime=0.01
  wires:
  Pulse Generator/1 -> I2C Reset/Trigger, I2C Reinitialisierung/Trigger

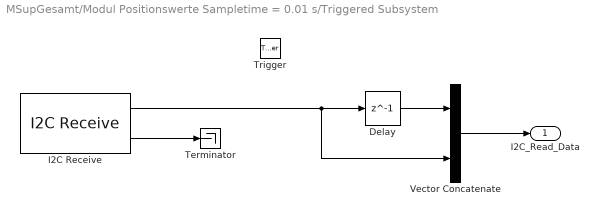
== system MSupGesamt/Modul Positionswerte Sampletime = 0.01 s/Triggered Subsystem ==
  Trigger : TriggerPort  TriggerType=function-call  VariantControl=(inherit)
  Delay : Delay  DelayLength=1  InitialCondition=0
  I2C Receive : c280xlib/I2C Receive  selectModule=I2C_A  addrFormat=7-Bit addressing  saSource=Specify via dialog  SAR=80  bitCount=8  dataLength=10  initValue=0  NACK=on  STP=off  STR=on  sampleTime=-1  dataType=uint8
      settings: SourceProductName=Embedded Coder Support Package for Texas Instruments C2000 Processors  SourceProductBaseCode=TIC2000
  Terminator : Terminator
  Vector Concatenate : Concatenate
  I2C_Read_Data : Outport
  wires:
  I2C Receive/2 -> Terminator/1
  I2C Receive/1 -> Vector Concatenate/2, Delay/1
  Delay/1 -> Vector Concatenate/1
  Vector Concatenate/1 -> I2C_Read_Data/1

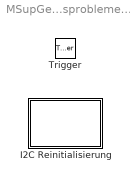
== system MSupGesamt/Modul Positionswerte Sampletime = 0.01 s/I2C Reset (behebt Stabilitätsprobleme der I2C-Verbindung)/I2C Reinitialisierung ==
  Trigger : TriggerPort  TriggerType=falling  VariantControl=(inherit)
  I2C Reinitialisierung : MATLAB Function  TreatAsAtomicUnit=on

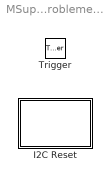
== system MSupGesamt/Modul Positionswerte Sampletime = 0.01 s/I2C Reset (behebt Stabilitätsprobleme der I2C-Verbindung)/I2C Reset ==
  Trigger : TriggerPort  VariantControl=(inherit)
  I2C Reset : MATLAB Function  TreatAsAtomicUnit=on

== stateflow chart MSupGesamt/Subsystem1/Sensoren ==
  state wartenkurz [commented out]
  state WartenKurz
  state warten5
    en:
    PWM_Out = 0;
  state warten [commented out]
    en:
    PWM_Out = 0;
  state warten3 [commented out]
  state Zeiger_im_Weg
    PWM_Out = 80;
    richtung = 0;
  state Sensor_frei
  state SchwarzOderBunt [commented out]
  state Schwarz [commented out]
    PWM_Out = 80;
    richtung = 0;
  state Farbe [commented out]
  state WuerfelOderZylinder
  state blau [commented out]
    en:
    farbenStatus = 0;
  state rot [commented out]
    en:
    farbenStatus = 1;
  state Zylinder
    PWM_Out = 80;
    richtung = 0;
  state Wuerfel
  state Blau
    en:
    farbenStatus = 0;
  state Rot
    en:
    farbenStatus = 1;
  state warten4 [commented out]
  state Warten
  state Bunt [commented out]
    PWM_Out = 80;
    richtung = 1;
  state Wuerfl
    PWM_Out = 80;
    richtung = 1;
  Bunt -> wartenkurz [commented out] : [licht ==1]
  Schwarz -> wartenkurz [commented out] : [licht == 1]
  Zylinder -> WartenKurz : [licht == 1]
  Wuerfl -> WartenKurz : [licht == 1]
  wartenkurz -> warten [commented out] : after(1,msec)
  WartenKurz -> warten5 : after(1,msec)
  (default) -> warten5
  (default) -> warten [commented out]
  Zeiger_im_Weg -> warten5 : after(1,msec)
  warten5 -> Zeiger_im_Weg [order 1] : [licht == 1 && farbe > 300]
  warten5 -> Sensor_frei [order 2] : [licht == 0]
  warten -> warten3 [commented out] : [licht == 0]
  warten3 -> SchwarzOderBunt [commented out] : after(0.5,sec)
  Sensor_frei -> WuerfelOderZylinder : after(0.5,sec)
  SchwarzOderBunt -> Schwarz [commented out] : [farbe > 2380]
  SchwarzOderBunt -> Farbe [commented out] : [farbe < 2380]
  Farbe -> blau [commented out] : [farbe > 1500]
  Farbe -> rot [commented out] : [farbe < 1500]
  WuerfelOderZylinder -> Zylinder [order 1] : [farbe > 2380]
  WuerfelOderZylinder -> Wuerfel [order 2] : [farbe < 2380]
  Wuerfel -> Blau [order 1] : [farbe > 1500]
  Wuerfel -> Rot [order 2] : [farbe < 1500]
  rot -> warten4 [commented out]
  blau -> warten4 [commented out]
  Blau -> Warten
  Rot -> Warten
  warten4 -> Bunt [commented out] : [weicheCheck == 0]
  Warten -> Wuerfl : [weicheCheck == 0]
  data: licht input; PWM_Out output; richtung output; farbenStatus output; farbe input; weicheCheck input

== stateflow chart MSupGesamt/Subsystem/Fahrt Modi ==
  state LinksDrehen
    entry:
    PWM_1_L = -drehGes;
    PWM_2_R = drehGes;
  state RechtsDrehen
    entry:
    PWM_1_L = drehGes;
    PWM_2_R = -drehGes;
  state Stehen
    entry:
    PWM_1_L = 0;
    PWM_2_R = 0;
  state GeradeausFahren
    entry:
    PWM_1_L = normalGes;
    PWM_2_R = normalGes;
  state Rueckwaerts
    entry:
    PWM_1_L = -drehGes;
    PWM_2_R = -drehGes;
  LinksDrehen -> RechtsDrehen [order 2] : [winkel < -10]
  RechtsDrehen -> LinksDrehen [order 2] : [winkel > 10]
  LinksDrehen -> Stehen [order 1] : [(winkel > -10 & winkel <10)||stop == 1||distanz < 300]
  Stehen -> LinksDrehen [order 2] : [winkel > 10 & stop==0]
  RechtsDrehen -> Stehen [order 1] : [(winkel > -10 & winkel < 10) || stop == 1||distanz < 300 ]
  Stehen -> RechtsDrehen [order 3] : [winkel < -10 & stop==0]
  (default) -> Stehen
  GeradeausFahren -> Stehen : [winkel < -10 || winkel > 10|| stop==1]
  Stehen -> GeradeausFahren [order 1] : [winkel > -10 & winkel < 10 & stop == 0 & rueck ==0]
  Stehen -> Rueckwaerts [order 4] : [winkel > -10 & winkel < 10 & stop == 0 & rueck == 1]
  Rueckwaerts -> Stehen : [winkel < -10 || winkel > 10|| stop==1]
  data: PWM_1_L output; PWM_2_R output; distanz input; winkel input; normalGes input; drehGes input; stop input; rueck input

== stateflow chart MSupGesamt/Chart ==
  state warten
    en:
    kill =1;
  state Anfang
    en:
    kill = 1;
  state Ende
    en:
    kill = 0;
  (default) -> warten
  warten -> Anfang : [start == 1]
  Anfang -> Ende : [finish == 1]
  Anfang -> Ende [commented out] : after(175,sec)
  data: start input int32; kill output; finish input

== matlab function MSupGesamt/Subsystem/Richtungs Wechsel M1  ==
  data: u input; y output
function y = fcn(u)
if u > 0
    y = 0;
else
    y = 1;
end

== matlab function MSupGesamt/Subsystem/Richtungs Wechsel M2 ==
  data: u input; y output
function y = fcn(u)
if u > 0
    y = 0;
else
    y = 1;
end

== stateflow chart MSupGesamt/Subsystem/Strecken Koordinaten ==
  state Position1
    entry:
    x_soll = 8036;
    y_soll = 3476;
    stop = 0;
    rueck = 0;
    finish = 0;
    uebergabe = 0;
  state Position7 [commented out]
    entry:
    x_soll = 10350;
    y_soll = 1280;
    stop = 0;
    rueck = 0;
  state Position9 [commented out]
    entry:
    x_soll = 8562;
    y_soll = 2931;
    stop = 0;
    rueck = 0;
  state Position10 [commented out]
    entry:
    x_soll = 8543;
    y_soll = 5772;
    stop = 0;
    rueck = 0;
  state Position11 [commented out]
    entry:
    x_soll = 8012;
    y_soll = 7945;
    stop = 0;
    rueck = 0;
  state Position12 [commented out]
    entry:
    x_soll = 5826;
    y_soll = 8762;
    stop = 0;
    rueck = 0;
  state Position14 [commented out]
    entry:
    x_soll = 3433;
    y_soll = 3592;
    stop = 0;
    rueck = 0;
  state Position13 [commented out]
    entry:
    x_soll = 8360;
    y_soll = 6442;
    stop = 0;
    rueck = 0;
  state Position16 [commented out]
    entry:
    x_soll = 10029;
    y_soll = 2391;
    stop = 0;
    rueck = 0;
  state Position15 [commented out]
    entry:
    x_soll = 4102;
    y_soll = 8250;
    stop = 0;
    rueck = 0;
  state Position20 [commented out]
    entry:
    x_soll = 3850;
    y_soll = 7700;
    stop = 0;
    rueck = 0;
  state Position19 [commented out]
    entry:
    x_soll = 3645;
    y_soll = 7338;
    stop = 0;
    rueck = 0;
  state Position8 [commented out]
    entry:
    x_soll = 12700;
    y_soll = -809;
    stop = 0;
    rueck = 0;
  state Position5 [commented out]
    entry:
    x_soll = 12800;
    y_soll = 324;
    stop = 0;
    rueck = 1;
  state Position6 [commented out]
    entry:
    x_soll = 12700;
    y_soll = -320;
    stop = 0;
    rueck = 0;
  state Position17 [commented out]
    entry:
    x_soll = 11031;
    y_soll = -1424;
    stop = 0;
    rueck = 0;
  state Position18 [commented out]
    entry:
    x_soll = 8738;
    y_soll = -1737;
    stop = 0;
    rueck = 0;
  state Stop
    entry:
    stop = 1;
    finish = 1;
  state Uebergabe [commented out]
    entry:
    uebergabe = 1;
    stop = 1;
    exit:
    uebergabe = 0;
  state Position21
    entry:
    x_soll = 10029;
    y_soll = 2391;
    stop = 0;
    rueck = 0;
  (default) -> Position1
  Position1 -> Position7 [commented out] : [ziel == 1]
  Position7 -> Position9 [commented out] : [ziel == 1]
  Position9 -> Position10 [commented out] : [ziel == 1]
  Position10 -> Position11 [commented out] : [ziel == 1]
  Position11 -> Position12 [commented out] : [ziel == 1]
  Position12 -> Position15 [commented out] : [ziel == 1]
  Position1 -> Position21 : [ziel == 1]
  Position19 -> Position14 [commented out] : [ziel == 1]
  Position20 -> Position19 [commented out] : [ziel == 1]
  Position15 -> Position20 [commented out] : [ziel == 1]
  Position14 -> Position13 [commented out] : [ziel == 1]
  Position13 -> Position16 [commented out] : [ziel == 1]
  Position16 -> Position8 [commented out] : [ziel == 1]
  Position17 -> Position18 [commented out] : [ziel == 1]
  Position5 -> Uebergabe [commented out] : [ziel == 1]
  Position18 -> Stop [commented out] : [ziel == 1]
  Position6 -> Position17 [commented out] : [ziel == 1]
  Position8 -> Position5 [commented out] : [ziel == 1]
  Uebergabe -> Position6 [commented out] : [angekommen == 1]
  Position21 -> Stop : [ziel == 1]
  data: x_soll output; y_soll output; ziel input; stop output; rueck output; finish output; uebergabe output; angekommen input

== matlab function MSupGesamt/Subsystem/Winkel und Distanz ==
  data: x_soll input; distanz output; y_soll input; x_ist input; y_ist input; alpha_ist input; winkel output; ziel output; rueck input
function [distanz, winkel, ziel] = fcn(x_soll, y_soll, x_ist, y_ist, alpha_ist, rueck)
    
    % Realtive Position der Ziel Koordinaten
    x_dif = x_soll - x_ist;
    y_dif = y_soll - y_ist;
    distanz = sqrt(x_dif^2 + y_dif^2);
    winkelVor = rad2deg(atan(y_dif/x_dif));
    
    % Drehwinkel Bestimmung
    if x_dif < 0
        winkelVor = winkelVor + 180;
    else
        if y_dif < 0
            winkelVor = winkelVor + 360;
        end
    end
    % Rückwärts Funktion
    if rueck == 1
        winkelVor = winkelVor + 180;
        if winkelVor > 360
            winkelVor = winkelVor -360;
        end
    end
    
    % rechnet aktuellen Winkel mit ein
    winkelVor = winkelVor - alpha_ist/10;
    
    % bestimmt kürzere Drehdistanz
    if winkelVor > 175 
        winkelVor = winkelVor - 360;
    end
    % Winkel wird ausgegebn
    winkel = winkelVor; 
    
    % checkt ob die nächste Koordinate angefahren werden kann
    if distanz < 300
        ziel = 1;
    else
        ziel = 0;
    end

== stateflow chart MSupGesamt/Subsystem1/Weichen Steuerung ==
  state linksdrehen
    en:
    PWM_Out = 50;
    DIR = 0;
    weicheCheck = 1;
  state blau
    en:
    weicheCheck = 0;
    PWM_Out = 0;
  state rot
    en:
    weicheCheck = 0;
    PWM_Out = 0;
  state rechtsdrehen
    en:
    PWM_Out = 50;
    DIR = 1;
    weicheCheck = 1;
  linksdrehen -> blau : after(0.19,sec)
  rot -> linksdrehen : [farbenStatus == 0]
  (default) -> blau
  blau -> rechtsdrehen : [farbenStatus == 1]
  rechtsdrehen -> rot : after(0.19,sec)
  data: farbenStatus input; PWM_Out output; DIR output; weicheCheck output single

== stateflow chart MSupGesamt/Subsystem2/Chart ==
  state warten
    en:
    PWM_Out = 0;
    DIR = 0;
    angekommen = 0;
  state hochFahren
    en:
    PWM_Out = 100;
    DIR = 0;
  state oben
    en:
    PWM_Out = 0;
    DIR = 0;
  state runterFahren
    en:
    PWM_Out = 100;
    DIR = 1;
    angekommen = 1;
  state unten
    en:
    PWM_Out = 0;
    DIR = 0;
  (default) -> warten
  warten -> hochFahren : [uebergabe == 1]
  hochFahren -> oben : [oben == 1]
  oben -> runterFahren : after(5,sec)
  runterFahren -> unten : [unten == 1]
  data: uebergabe input; PWM_Out output; DIR output; oben input; unten input; angekommen output

== stateflow chart MSupGesamt/Modul Positionswerte Sampletime = 0.01 s/Chart1 ==
  state Daten_einlesen
  state x0
  state x1_1
    entry: int16z_bin[0] = int8z_1[0];
    int16z_bin[1] = int8z_1[1];
    int16z_bin[2] = int8z_1[2];
    int16z_bin[3] = int8z_1[3];
    int16z_bin[4] = int8z_1[4];
    int16z_bin[5] = int8z_1[5]
    int16z_bin[6] = int8z_1[6];
    int16z_bin[7] = int8z_1[7];
    int16z_bin[8] = int8z_2[0];
    int16z_bin[9] = int8z_2[1];
    int16z_bin[10] = int8z_2[2];
    int16z_bin[11] = int8z_2[3];
    int16z_bin[12] = int8z_2[4];
    int16z_bin[13] = int8z_2[5]
    int16z_bin[14] = int8z_2[6];
    int16z_bin[15] = int8z_2[7];
  x0 -> Daten_einlesen
  (default) -> x0
  Daten_einlesen -> x1_1
  x1_1 -> Daten_einlesen
  data: int8z_1 input size=8; int8z_2 input size=8; int16z_bin output size=16 =0

== stateflow chart MSupGesamt/Modul Positionswerte Sampletime = 0.01 s/Chart2 ==
  state Daten_einlesen
  state x0
  state x1_1
    entry: int16y_bin[0] = int8y_1[0];
    int16y_bin[1] = int8y_1[1];
    int16y_bin[2] = int8y_1[2];
    int16y_bin[3] = int8y_1[3];
    int16y_bin[4] = int8y_1[4];
    int16y_bin[5] = int8y_1[5]
    int16y_bin[6] = int8y_1[6];
    int16y_bin[7] = int8y_1[7];
    int16y_bin[8] = int8y_2[0];
    int16y_bin[9] = int8y_2[1];
    int16y_bin[10] = int8y_2[2];
    int16y_bin[11] = int8y_2[3];
    int16y_bin[12] = int8y_2[4];
    int16y_bin[13] = int8y_2[5]
    int16y_bin[14] = int8y_2[6];
    int16y_bin[15] = int8y_2[7];
  x0 -> Daten_einlesen
  (default) -> x0
  Daten_einlesen -> x1_1
  x1_1 -> Daten_einlesen
  data: int8y_1 input size=8; int8y_2 input size=8; int16y_bin output size=16 =0

== stateflow chart MSupGesamt/Modul Positionswerte Sampletime = 0.01 s/Chart4 ==
  state Daten_einlesen
  state x0
  state x1_1
    entry: int16a1_bin[0] = int8a1_1[0];
    int16a1_bin[1] = int8a1_1[1];
    int16a1_bin[2] = int8a1_1[2];
    int16a1_bin[3] = int8a1_1[3];
    int16a1_bin[4] = int8a1_1[4];
    int16a1_bin[5] = int8a1_1[5]
    int16a1_bin[6] = int8a1_1[6];
    int16a1_bin[7] = int8a1_1[7];
    int16a1_bin[8] = int8a1_2[0];
    int16a1_bin[9] = int8a1_2[1];
    int16a1_bin[10] = int8a1_2[2];
    int16a1_bin[11] = int8a1_2[3];
    int16a1_bin[12] = int8a1_2[4];
    int16a1_bin[13] = int8a1_2[5]
    int16a1_bin[14] = int8a1_2[6];
    int16a1_bin[15] = int8a1_2[7];
  x0 -> Daten_einlesen
  (default) -> x0
  Daten_einlesen -> x1_1
  x1_1 -> Daten_einlesen
  data: int8a1_1 input size=8; int8a1_2 input size=8; int16a1_bin output size=16 =0

== stateflow chart MSupGesamt/Modul Positionswerte Sampletime = 0.01 s/Chart6 ==
  state Daten_einlesen
  state x0
  state x1_1
    entry: int16x_bin[0] = int8x_1[0];
    int16x_bin[1] = int8x_1[1];
    int16x_bin[2] = int8x_1[2];
    int16x_bin[3] = int8x_1[3];
    int16x_bin[4] = int8x_1[4];
    int16x_bin[5] = int8x_1[5]
    int16x_bin[6] = int8x_1[6];
    int16x_bin[7] = int8x_1[7];
    int16x_bin[8] = int8x_2[0];
    int16x_bin[9] = int8x_2[1];
    int16x_bin[10] = int8x_2[2];
    int16x_bin[11] = int8x_2[3];
    int16x_bin[12] = int8x_2[4];
    int16x_bin[13] = int8x_2[5]
    int16x_bin[14] = int8x_2[6];
    int16x_bin[15] = int8x_2[7];
  x0 -> Daten_einlesen
  (default) -> x0
  Daten_einlesen -> x1_1
  x1_1 -> Daten_einlesen
  data: int8x_1 input size=8; int8x_2 input size=8; int16x_bin output size=16 =0
